simulink model "DriveSystemControl"  (R2023b)
settings: Solver=FixedStepAuto  StartTime=0.0  StopTime=Inf  FixedStep=0.001  RelTol=1e-3
PostLoadFcn:
  | if any(exist('dsrtsu_mdlpostloadfcn', 'file') ~= 0), dsrtsu_mdlpostloadfcn('Execute', bdroot); end
InitFcn:
  | , if any(exist('rtifpga_mdlclblib', 'file') ~= 0), rtifpga_mdlclblib('Init', bdroot); end,
  | , if any(exist('dsmpb_private', 'file') ~= 0), dsmpb_private('dsmpb_mdlclblib', 'Init', bdroot); end,
libraries: dsmpblib x2
(part 11 of 11)

== system DriveSystemControl/Bus Configuration (1) - Out/Simulated ECUs/Virya Controller CAN File 08082024/Telematics/RX/PDUs/TCU03/sigControllerOverCurrent/ISignal Value ==
  ISignal Value : Inport
  Term_sigControllerOverCurrent Value : Terminator
  _ISignal Value_ : BusSelector  OutputSignals=sigControllerOverCurrent Value
  wires:
  ISignal Value/1 -> _ISignal Value_/1  "ISignal Value"
  _ISignal Value_/1 -> Term_sigControllerOverCurrent Value/1  "<sigControllerOverCurrent Value>"

== system DriveSystemControl/Bus Configuration (1) - Out/Simulated ECUs/Virya Controller CAN File 08082024/Telematics/RX/PDUs/TCU03/sigControllerOvertempCutback/ISignal Value ==
  ISignal Value : Inport
  Term_sigControllerOvertempCutback Value : Terminator
  _ISignal Value_ : BusSelector  OutputSignals=sigControllerOvertempCutback Value
  wires:
  ISignal Value/1 -> _ISignal Value_/1  "ISignal Value"
  _ISignal Value_/1 -> Term_sigControllerOvertempCutback Value/1  "<sigControllerOvertempCutback Value>"

== system DriveSystemControl/Bus Configuration (1) - Out/Simulated ECUs/Virya Controller CAN File 08082024/Telematics/RX/PDUs/TCU03/sigControllerSevereOvertemp/ISignal Value ==
  ISignal Value : Inport
  Term_sigControllerSevereOvertemp Value : Terminator
  _ISignal Value_ : BusSelector  OutputSignals=sigControllerSevereOvertemp Value
  wires:
  ISignal Value/1 -> _ISignal Value_/1  "ISignal Value"
  _ISignal Value_/1 -> Term_sigControllerSevereOvertemp Value/1  "<sigControllerSevereOvertemp Value>"

== system DriveSystemControl/Bus Configuration (1) - Out/Simulated ECUs/Virya Controller CAN File 08082024/Telematics/RX/PDUs/TCU03/sigControllerSevereUndertemp/ISignal Value ==
  ISignal Value : Inport
  Term_sigControllerSevereUndertemp Value : Terminator
  _ISignal Value_ : BusSelector  OutputSignals=sigControllerSevereUndertemp Value
  wires:
  ISignal Value/1 -> _ISignal Value_/1  "ISignal Value"
  _ISignal Value_/1 -> Term_sigControllerSevereUndertemp Value/1  "<sigControllerSevereUndertemp Value>"

== system DriveSystemControl/Bus Configuration (1) - Out/Simulated ECUs/Virya Controller CAN File 08082024/Telematics/RX/PDUs/TCU03/sigCurrentSensorFault/ISignal Value ==
  ISignal Value : Inport
  Term_sigCurrentSensorFault Value : Terminator
  _ISignal Value_ : BusSelector  OutputSignals=sigCurrentSensorFault Value
  wires:
  ISignal Value/1 -> _ISignal Value_/1  "ISignal Value"
  _ISignal Value_/1 -> Term_sigCurrentSensorFault Value/1  "<sigCurrentSensorFault Value>"

== system DriveSystemControl/Bus Configuration (1) - Out/Simulated ECUs/Virya Controller CAN File 08082024/Telematics/RX/PDUs/TCU03/sigEEPROMFailure/ISignal Value ==
  ISignal Value : Inport
  Term_sigEEPROMFailure Value : Terminator
  _ISignal Value_ : BusSelector  OutputSignals=sigEEPROMFailure Value
  wires:
  ISignal Value/1 -> _ISignal Value_/1  "ISignal Value"
  _ISignal Value_/1 -> Term_sigEEPROMFailure Value/1  "<sigEEPROMFailure Value>"

== system DriveSystemControl/Bus Configuration (1) - Out/Simulated ECUs/Virya Controller CAN File 08082024/Telematics/RX/PDUs/TCU03/sigHighPedalDisable/ISignal Value ==
  ISignal Value : Inport
  Term_sigHighPedalDisable Value : Terminator
  _ISignal Value_ : BusSelector  OutputSignals=sigHighPedalDisable Value
  wires:
  ISignal Value/1 -> _ISignal Value_/1  "ISignal Value"
  _ISignal Value_/1 -> Term_sigHighPedalDisable Value/1  "<sigHighPedalDisable Value>"

== system DriveSystemControl/Bus Configuration (1) - Out/Simulated ECUs/Virya Controller CAN File 08082024/Telematics/RX/PDUs/TCU03/sigInsulationResistanceLow/ISignal Value ==
  ISignal Value : Inport
  Term_sigInsulationResistanceLow Value : Terminator
  _ISignal Value_ : BusSelector  OutputSignals=sigInsulationResistanceLow Value
  wires:
  ISignal Value/1 -> _ISignal Value_/1  "ISignal Value"
  _ISignal Value_/1 -> Term_sigInsulationResistanceLow Value/1  "<sigInsulationResistanceLow Value>"

== system DriveSystemControl/Bus Configuration (1) - Out/Simulated ECUs/Virya Controller CAN File 08082024/Telematics/RX/PDUs/TCU03/sigMainContactorWelded/ISignal Value ==
  ISignal Value : Inport
  Term_sigMainContactorWelded Value : Terminator
  _ISignal Value_ : BusSelector  OutputSignals=sigMainContactorWelded Value
  wires:
  ISignal Value/1 -> _ISignal Value_/1  "ISignal Value"
  _ISignal Value_/1 -> Term_sigMainContactorWelded Value/1  "<sigMainContactorWelded Value>"

== system DriveSystemControl/Bus Configuration (1) - Out/Simulated ECUs/Virya Controller CAN File 08082024/Telematics/RX/PDUs/TCU03/sigMainContactordidnotClose/ISignal Value ==
  ISignal Value : Inport
  Term_sigMainContactordidnotClose Value : Terminator
  _ISignal Value_ : BusSelector  OutputSignals=sigMainContactordidnotClose Value
  wires:
  ISignal Value/1 -> _ISignal Value_/1  "ISignal Value"
  _ISignal Value_/1 -> Term_sigMainContactordidnotClose Value/1  "<sigMainContactordidnotClose Value>"

== system DriveSystemControl/Bus Configuration (1) - Out/Simulated ECUs/Virya Controller CAN File 08082024/Telematics/RX/PDUs/TCU03/sigMainOpenShort/ISignal Value ==
  ISignal Value : Inport
  Term_sigMainOpenShort Value : Terminator
  _ISignal Value_ : BusSelector  OutputSignals=sigMainOpenShort Value
  wires:
  ISignal Value/1 -> _ISignal Value_/1  "ISignal Value"
  _ISignal Value_/1 -> Term_sigMainOpenShort Value/1  "<sigMainOpenShort Value>"

== system DriveSystemControl/Bus Configuration (1) - Out/Simulated ECUs/Virya Controller CAN File 08082024/Telematics/RX/PDUs/TCU03/sigMotorCharacterization/ISignal Value ==
  ISignal Value : Inport
  Term_sigMotorCharacterization Value : Terminator
  _ISignal Value_ : BusSelector  OutputSignals=sigMotorCharacterization Value
  wires:
  ISignal Value/1 -> _ISignal Value_/1  "ISignal Value"
  _ISignal Value_/1 -> Term_sigMotorCharacterization Value/1  "<sigMotorCharacterization Value>"

== system DriveSystemControl/Bus Configuration (1) - Out/Simulated ECUs/Virya Controller CAN File 08082024/Telematics/RX/PDUs/TCU03/sigMotorPhaseOpen/ISignal Value ==
  ISignal Value : Inport
  Term_sigMotorPhaseOpen Value : Terminator
  _ISignal Value_ : BusSelector  OutputSignals=sigMotorPhaseOpen Value
  wires:
  ISignal Value/1 -> _ISignal Value_/1  "ISignal Value"
  _ISignal Value_/1 -> Term_sigMotorPhaseOpen Value/1  "<sigMotorPhaseOpen Value>"

== system DriveSystemControl/Bus Configuration (1) - Out/Simulated ECUs/Virya Controller CAN File 08082024/Telematics/RX/PDUs/TCU03/sigMotorTempHotCutback/ISignal Value ==
  ISignal Value : Inport
  Term_sigMotorTempHotCutback Value : Terminator
  _ISignal Value_ : BusSelector  OutputSignals=sigMotorTempHotCutback Value
  wires:
  ISignal Value/1 -> _ISignal Value_/1  "ISignal Value"
  _ISignal Value_/1 -> Term_sigMotorTempHotCutback Value/1  "<sigMotorTempHotCutback Value>"

== system DriveSystemControl/Bus Configuration (1) - Out/Simulated ECUs/Virya Controller CAN File 08082024/Telematics/RX/PDUs/TCU03/sigMotorTempSensorFault/ISignal Value ==
  ISignal Value : Inport
  Term_sigMotorTempSensorFault Value : Terminator
  _ISignal Value_ : BusSelector  OutputSignals=sigMotorTempSensorFault Value
  wires:
  ISignal Value/1 -> _ISignal Value_/1  "ISignal Value"
  _ISignal Value_/1 -> Term_sigMotorTempSensorFault Value/1  "<sigMotorTempSensorFault Value>"

== system DriveSystemControl/Bus Configuration (1) - Out/Simulated ECUs/Virya Controller CAN File 08082024/Telematics/RX/PDUs/TCU03/sigOEM_BatterySTOPSignal/ISignal Value ==
  ISignal Value : Inport
  Term_sigOEM_BatterySTOPSignal Value : Terminator
  _ISignal Value_ : BusSelector  OutputSignals=sigOEM_BatterySTOPSignal Value
  wires:
  ISignal Value/1 -> _ISignal Value_/1  "ISignal Value"
  _ISignal Value_/1 -> Term_sigOEM_BatterySTOPSignal Value/1  "<sigOEM_BatterySTOPSignal Value>"

== system DriveSystemControl/Bus Configuration (1) - Out/Simulated ECUs/Virya Controller CAN File 08082024/Telematics/RX/PDUs/TCU03/sigOEM_NoBatteryCAN/ISignal Value ==
  ISignal Value : Inport
  Term_sigOEM_NoBatteryCAN Value : Terminator
  _ISignal Value_ : BusSelector  OutputSignals=sigOEM_NoBatteryCAN Value
  wires:
  ISignal Value/1 -> _ISignal Value_/1  "ISignal Value"
  _ISignal Value_/1 -> Term_sigOEM_NoBatteryCAN Value/1  "<sigOEM_NoBatteryCAN Value>"

== system DriveSystemControl/Bus Configuration (1) - Out/Simulated ECUs/Virya Controller CAN File 08082024/Telematics/RX/PDUs/TCU03/sigOSGeneral/ISignal Value ==
  ISignal Value : Inport
  Term_sigOSGeneral Value : Terminator
  _ISignal Value_ : BusSelector  OutputSignals=sigOSGeneral Value
  wires:
  ISignal Value/1 -> _ISignal Value_/1  "ISignal Value"
  _ISignal Value_/1 -> Term_sigOSGeneral Value/1  "<sigOSGeneral Value>"

== system DriveSystemControl/Bus Configuration (1) - Out/Simulated ECUs/Virya Controller CAN File 08082024/Telematics/RX/PDUs/TCU03/sigPMACCommissioningNeeded/ISignal Value ==
  ISignal Value : Inport
  Term_sigPMACCommissioningNeeded Value : Terminator
  _ISignal Value_ : BusSelector  OutputSignals=sigPMACCommissioningNeeded Value
  wires:
  ISignal Value/1 -> _ISignal Value_/1  "ISignal Value"
  _ISignal Value_/1 -> Term_sigPMACCommissioningNeeded Value/1  "<sigPMACCommissioningNeeded Value>"

== system DriveSystemControl/Bus Configuration (1) - Out/Simulated ECUs/Virya Controller CAN File 08082024/Telematics/RX/PDUs/TCU03/sigParameterChangeFault/ISignal Value ==
  ISignal Value : Inport
  Term_sigParameterChangeFault Value : Terminator
  _ISignal Value_ : BusSelector  OutputSignals=sigParameterChangeFault Value
  wires:
  ISignal Value/1 -> _ISignal Value_/1  "ISignal Value"
  _ISignal Value_/1 -> Term_sigParameterChangeFault Value/1  "<sigParameterChangeFault Value>"

== system DriveSystemControl/Bus Configuration (1) - Out/Simulated ECUs/Virya Controller CAN File 08082024/Telematics/RX/PDUs/TCU03/sigPhasePWMMismatch/ISignal Value ==
  ISignal Value : Inport
  Term_sigPhasePWMMismatch Value : Terminator
  _ISignal Value_ : BusSelector  OutputSignals=sigPhasePWMMismatch Value
  wires:
  ISignal Value/1 -> _ISignal Value_/1  "ISignal Value"
  _ISignal Value_/1 -> Term_sigPhasePWMMismatch Value/1  "<sigPhasePWMMismatch Value>"

== system DriveSystemControl/Bus Configuration (1) - Out/Simulated ECUs/Virya Controller CAN File 08082024/Telematics/RX/PDUs/TCU03/sigPrechargeFailed/ISignal Value ==
  ISignal Value : Inport
  Term_sigPrechargeFailed Value : Terminator
  _ISignal Value_ : BusSelector  OutputSignals=sigPrechargeFailed Value
  wires:
  ISignal Value/1 -> _ISignal Value_/1  "ISignal Value"
  _ISignal Value_/1 -> Term_sigPrechargeFailed Value/1  "<sigPrechargeFailed Value>"

== system DriveSystemControl/Bus Configuration (1) - Out/Simulated ECUs/Virya Controller CAN File 08082024/Telematics/RX/PDUs/TCU03/sigSevereBPosOvervoltage/ISignal Value ==
  ISignal Value : Inport
  Term_sigSevereBPosOvervoltage Value : Terminator
  _ISignal Value_ : BusSelector  OutputSignals=sigSevereBPosOvervoltage Value
  wires:
  ISignal Value/1 -> _ISignal Value_/1  "ISignal Value"
  _ISignal Value_/1 -> Term_sigSevereBPosOvervoltage Value/1  "<sigSevereBPosOvervoltage Value>"

== system DriveSystemControl/Bus Configuration (1) - Out/Simulated ECUs/Virya Controller CAN File 08082024/Telematics/RX/PDUs/TCU03/sigSevereBPosUndervoltage/ISignal Value ==
  ISignal Value : Inport
  Term_sigSevereBPosUndervoltage Value : Terminator
  _ISignal Value_ : BusSelector  OutputSignals=sigSevereBPosUndervoltage Value
  wires:
  ISignal Value/1 -> _ISignal Value_/1  "ISignal Value"
  _ISignal Value_/1 -> Term_sigSevereBPosUndervoltage Value/1  "<sigSevereBPosUndervoltage Value>"

== system DriveSystemControl/Bus Configuration (1) - Out/Simulated ECUs/Virya Controller CAN File 08082024/Telematics/RX/PDUs/TCU03/sigSevereKSIOvervoltage/ISignal Value ==
  ISignal Value : Inport
  Term_sigSevereKSIOvervoltage Value : Terminator
  _ISignal Value_ : BusSelector  OutputSignals=sigSevereKSIOvervoltage Value
  wires:
  ISignal Value/1 -> _ISignal Value_/1  "ISignal Value"
  _ISignal Value_/1 -> Term_sigSevereKSIOvervoltage Value/1  "<sigSevereKSIOvervoltage Value>"

== system DriveSystemControl/Bus Configuration (1) - Out/Simulated ECUs/Virya Controller CAN File 08082024/Telematics/RX/PDUs/TCU03/sigSevereKSIUndervoltage/ISignal Value ==
  ISignal Value : Inport
  Term_sigSevereKSIUndervoltage Value : Terminator
  _ISignal Value_ : BusSelector  OutputSignals=sigSevereKSIUndervoltage Value
  wires:
  ISignal Value/1 -> _ISignal Value_/1  "ISignal Value"
  _ISignal Value_/1 -> Term_sigSevereKSIUndervoltage Value/1  "<sigSevereKSIUndervoltage Value>"

== system DriveSystemControl/Bus Configuration (1) - Out/Simulated ECUs/Virya Controller CAN File 08082024/Telematics/RX/PDUs/TCU03/sigSinCosMisalignment/ISignal Value ==
  ISignal Value : Inport
  Term_sigSinCosMisalignment Value : Terminator
  _ISignal Value_ : BusSelector  OutputSignals=sigSinCosMisalignment Value
  wires:
  ISignal Value/1 -> _ISignal Value_/1  "ISignal Value"
  _ISignal Value_/1 -> Term_sigSinCosMisalignment Value/1  "<sigSinCosMisalignment Value>"

== system DriveSystemControl/Bus Configuration (1) - Out/Simulated ECUs/Virya Controller CAN File 08082024/Telematics/RX/PDUs/TCU03/sigSinCosSensorFault/ISignal Value ==
  ISignal Value : Inport
  Term_sigSinCosSensorFault Value : Terminator
  _ISignal Value_ : BusSelector  OutputSignals=sigSinCosSensorFault Value
  wires:
  ISignal Value/1 -> _ISignal Value_/1  "ISignal Value"
  _ISignal Value_/1 -> Term_sigSinCosSensorFault Value/1  "<sigSinCosSensorFault Value>"

== system DriveSystemControl/Bus Configuration (1) - Out/Simulated ECUs/Virya Controller CAN File 08082024/Telematics/RX/PDUs/TCU03/sigStallDetected/ISignal Value ==
  ISignal Value : Inport
  Term_sigStallDetected Value : Terminator
  _ISignal Value_ : BusSelector  OutputSignals=sigStallDetected Value
  wires:
  ISignal Value/1 -> _ISignal Value_/1  "ISignal Value"
  _ISignal Value_/1 -> Term_sigStallDetected Value/1  "<sigStallDetected Value>"

== system DriveSystemControl/Bus Configuration (1) - Out/Simulated ECUs/Virya Controller CAN File 08082024/Telematics/RX/PDUs/TCU03/sigSupervisorFault/ISignal Value ==
  ISignal Value : Inport
  Term_sigSupervisorFault Value : Terminator
  _ISignal Value_ : BusSelector  OutputSignals=sigSupervisorFault Value
  wires:
  ISignal Value/1 -> _ISignal Value_/1  "ISignal Value"
  _ISignal Value_/1 -> Term_sigSupervisorFault Value/1  "<sigSupervisorFault Value>"

== system DriveSystemControl/Bus Configuration (1) - Out/Simulated ECUs/Virya Controller CAN File 08082024/Telematics/RX/PDUs/TCU03/sigThrottlewiperHigh/ISignal Value ==
  ISignal Value : Inport
  Term_sigThrottlewiperHigh Value : Terminator
  _ISignal Value_ : BusSelector  OutputSignals=sigThrottlewiperHigh Value
  wires:
  ISignal Value/1 -> _ISignal Value_/1  "ISignal Value"
  _ISignal Value_/1 -> Term_sigThrottlewiperHigh Value/1  "<sigThrottlewiperHigh Value>"

== system DriveSystemControl/Bus Configuration (1) - Out/Simulated ECUs/Virya Controller CAN File 08082024/Telematics/RX/PDUs/TCU03/sigThrottlewiperLow/ISignal Value ==
  ISignal Value : Inport
  Term_sigThrottlewiperLow Value : Terminator
  _ISignal Value_ : BusSelector  OutputSignals=sigThrottlewiperLow Value
  wires:
  ISignal Value/1 -> _ISignal Value_/1  "ISignal Value"
  _ISignal Value_/1 -> Term_sigThrottlewiperLow Value/1  "<sigThrottlewiperLow Value>"

== system DriveSystemControl/Bus Configuration (1) - Out/Simulated ECUs/Virya Controller CAN File 08082024/Telematics/RX/PDUs/TCU03/sigVCLRunTimeError/ISignal Value ==
  ISignal Value : Inport
  Term_sigVCLRunTimeError Value : Terminator
  _ISignal Value_ : BusSelector  OutputSignals=sigVCLRunTimeError Value
  wires:
  ISignal Value/1 -> _ISignal Value_/1  "ISignal Value"
  _ISignal Value_/1 -> Term_sigVCLRunTimeError Value/1  "<sigVCLRunTimeError Value>"

== system DriveSystemControl/Bus Configuration (1) - Out/Simulated ECUs/Virya Controller CAN File 08082024/Telematics/RX/PDUs/TCU04/sigMCU5_DriveMode/ISignal Value ==
  ISignal Value : Inport
  Term_sigMCU5_DriveMode Value : Terminator
  _ISignal Value_ : BusSelector  OutputSignals=sigMCU5_DriveMode Value
  wires:
  ISignal Value/1 -> _ISignal Value_/1  "ISignal Value"
  _ISignal Value_/1 -> Term_sigMCU5_DriveMode Value/1  "<sigMCU5_DriveMode Value>"

== system DriveSystemControl/Bus Configuration (1) - Out/Simulated ECUs/Virya Controller CAN File 08082024/Telematics/RX/PDUs/TCU04/sigMCU5_Efficiency/ISignal Value ==
  ISignal Value : Inport
  Term_sigMCU5_Efficiency Value : Terminator
  _ISignal Value_ : BusSelector  OutputSignals=sigMCU5_Efficiency Value
  wires:
  ISignal Value/1 -> _ISignal Value_/1  "ISignal Value"
  _ISignal Value_/1 -> Term_sigMCU5_Efficiency Value/1  "<sigMCU5_Efficiency Value>"

== system DriveSystemControl/Bus Configuration (1) - Out/Simulated ECUs/Virya Controller CAN File 08082024/Telematics/RX/PDUs/TCU04/sigMCU5_Hillhold/ISignal Value ==
  ISignal Value : Inport
  Term_sigMCU5_Hillhold Value : Terminator
  _ISignal Value_ : BusSelector  OutputSignals=sigMCU5_Hillhold Value
  wires:
  ISignal Value/1 -> _ISignal Value_/1  "ISignal Value"
  _ISignal Value_/1 -> Term_sigMCU5_Hillhold Value/1  "<sigMCU5_Hillhold Value>"

== system DriveSystemControl/Bus Configuration (1) - Out/Simulated ECUs/Virya Controller CAN File 08082024/Telematics/RX/PDUs/TCU04/sigMCU5_RegenFlag/ISignal Value ==
  ISignal Value : Inport
  Term_sigMCU5_RegenFlag Value : Terminator
  _ISignal Value_ : BusSelector  OutputSignals=sigMCU5_RegenFlag Value
  wires:
  ISignal Value/1 -> _ISignal Value_/1  "ISignal Value"
  _ISignal Value_/1 -> Term_sigMCU5_RegenFlag Value/1  "<sigMCU5_RegenFlag Value>"

== system DriveSystemControl/Bus Configuration (1) - Out/Simulated ECUs/Virya Controller CAN File 08082024/Telematics/RX/PDUs/TCU04/sigMCU5_Speed/ISignal Value ==
  ISignal Value : Inport
  Term_sigMCU5_Speed Value : Terminator
  _ISignal Value_ : BusSelector  OutputSignals=sigMCU5_Speed Value
  wires:
  ISignal Value/1 -> _ISignal Value_/1  "ISignal Value"
  _ISignal Value_/1 -> Term_sigMCU5_Speed Value/1  "<sigMCU5_Speed Value>"

== system DriveSystemControl/Bus Configuration (1) - Out/Simulated ECUs/Virya Controller CAN File 08082024/Telematics/RX/PDUs/TCU05/sigMCU6_Odometer/ISignal Value ==
  ISignal Value : Inport
  Term_sigMCU6_Odometer Value : Terminator
  _ISignal Value_ : BusSelector  OutputSignals=sigMCU6_Odometer Value
  wires:
  ISignal Value/1 -> _ISignal Value_/1  "ISignal Value"
  _ISignal Value_/1 -> Term_sigMCU6_Odometer Value/1  "<sigMCU6_Odometer Value>"
